simulink library "THBCreator"  (Simulink 8.2)
settings: Solver=ode45  StartTime=0.0  StopTime=10.0  RelTol=1e-3
settings Model: Creator=lena.frank  LastModifiedBy=drhf

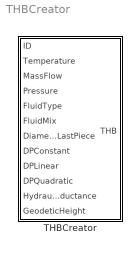
== system THBCreator ==
  THBCreator : Subsystem  InitFcn=load('THB.mat');  mask(THBCreator){Inport_ID=on, Inport_T=on, Inport_mdot=on, Inport_p=on, Inport_type=on, Inport_mix=on, Inport_d=on, Inport_c=on, Inport_l=on, Inport_q=on, Inport_LH=on, Inport_H=on, ID=20001, T=20, mdot=0, p=1e5, FluidType=1, FluidMix=0, d=0.01, c=0, l=0, q=0, LH=0, H=0, Annotation_ID=off, Annotation_T=off, Annotation_mdot=off, Annotation_p=off, Annotation_type=off, Annotation_mix=off, Annotation_d=off, Annotation_c=off, Annotation_l=off, Annotation_q=off, Annotation_LH=off, Annotation_H=off}
      mask prompts: Inport_ID "ID as inport"; Inport_T "temperature as inport"; Inport_mdot "mass flow rate as inport"; Inport_p "pressure as inport"; Inport_type "fluid type as inport"; Inport_mix "fluid mix as inport"; Inport_d "diameter last piece as inport"; Inport_c "constant pressure drop coefficient as inport"; Inport_l "linear pressure drop coefficient as inport"; Inport_q "quadratic pressure drop coefficient as inport"; Inport_LH "hydraulic inductance as inport"; Inport_H "geodetic height as inport"; ID "ID [1]"; T "temperature [°C]"; mdot "mass flow rate [kg/s]"; p "pressure [Pa]"; FluidType "fluid type [enum]"; FluidMix "fluid mix [1]"; d "diameter last piece [m]"; c "constant pressure drop coefficient [Pa]"; l "linear pressure drop coefficient [Pa/(kg/s)]"; q "quadratic pressure drop coefficient [Pa/(kg/s)²]"; LH "hydraulic inductance [1/m]"; H "geodetic height"; Annotation_ID "ID as annotation"; Annotation_T "temperature as annotation"; Annotation_mdot "mass flow rate as annotation"; Annotation_p "pressure as annotation"; Annotation_type "fluid type as annotation"; Annotation_mix "fluid mix as annotation"; Annotation_d "diameter last piece as annotation"; Annotation_c "constant pressure drop coefficient as annotation"; Annotation_l "linear pressure drop coefficient as annotation"; Annotation_q "quadratic pressure drop coefficient as annotation"; Annotation_LH "hydraulic inductance as annotation"; Annotation_H "geodetic height as annotation"
      mask help: This block creates a THB from input signals.
      mask init:
      | MaskValue = get_param(gcb,'MaskValues');
      |     
      | if strcmp(MaskValue{1},'on') %ID
      |     if ~strcmp(get_param([gcb,'/ID'],'BlockType'),'Inport')
      |         delete_line(gcb,'ID/1','BusCreator/1'); %delete connection
      |         delete_block([gcb,'/ID']); %delete block
      |         add_block('built-in/Inport',[gcb,'/ID']); %add new block
      |         set_param([gcb, '/ID'],'Position',[50   1*50+8   50+30   1*50+8+14]); %set new block's position
      |         add_line(gcb,'ID/1','BusCreator/1'); %add new connection
      |         handles=get_param([gcb, '/ID'],'LineHandles'); %get line handles
      |         set(handles.Outport(1),'Name','ID'); %set line name
      |     end
      | else
      |     if ~strcmp(get_param([gcb,'/ID'],'BlockType'),'Constant')
      |         delete_line(gcb,'ID/1','BusCreator/1'); %delete connection
      |         delete_block([gcb,'/ID']); %delete block
      |         add_block('built-in/Constant',[gcb,'/ID']); %add new block
      |         set_param([gcb, '/ID'],'Position',[50   1*50   50+30   1*50+30]); %set new block's position
      |         set_param([gcb, '/ID'],'Value','ID'); %set mask varible as value
      |         add_line(gcb,'ID/1','BusCreator/1'); %add new connection
      |         handles=get_param([gcb, '/ID'],'LineHandles'); %get line handles
      |         set(handles.Outport(1),'Name','ID'); %set line name
      |     end
      | end
      | 
      | if strcmp(MaskValue{2},'on') %T
      |     if ~strcmp(get_param([gcb,'/Temperature'],'BlockType'),'Inport')
      |         delete_line(gcb,'Temperature/1','BusCreator/2'); %delete connection
      |         delete_block([gcb,'/Temperature']); %delete block
      |         add_block('built-in/Inport',[gcb,'/Temperature']); %add new block
      |         set_param([gcb, '/Temperature'],'Position',[50   2*50+8   50+30   2*50+8+14]); %set new block's position
      |         add_line(gcb,'Temperature/1','BusCreator/2'); %add new connection
      |         handles=get_param([gcb, '/Temperature'],'LineHandles'); %get line handles
      |         set(handles.Outport(1),'Name','Temperature'); %set line name
      |     end
      | else
      |     if ~strcmp(get_param([gcb,'/Temperature'],'BlockType'),'Constant')
      |         delete_line(gcb,'Temperature/1','BusCreator/2'); %delete connection
      |         delete_block([gcb,'/Temperature']); %delete block
      |         add_block('built-in/Constant',[gcb,'/Temperature']); %add new block
      |         set_param([gcb, '/Temperature'],'Position',[50   2*50   50+30   2*50+30]); %set new block's position
      |         set_param([gcb, '/Temperature'],'Value','T'); %set mask varible as value
      |         add_line(gcb,'Temperature/1','BusCreator/2'); %add new connection
      |         handles=get_param([gcb, '/Temperature'],'LineHandles'); %get line handles
      |         set(handles.Outport(1),'Name','Temperature'); %set line name
      |     end
      | end
      | 
      | if strcmp(MaskValue{3},'on') %MassFlow
      |     if ~strcmp(get_param([gcb,'/MassFlow'],'BlockType'),'Inport')
      |         delete_line(gcb,'MassFlow/1','BusCreator/3'); %delete connection
      |         delete_block([gcb,'/MassFlow']); %delete block
      |         add_block('built-in/Inport',[gcb,'/MassFlow']); %add new block
      |         set_param([gcb, '/MassFlow'],'Position',[50   3*50+8   50+30   3*50+8+14]); %set new block's position
      |         add_line(gcb,'MassFlow/1','BusCreator/3'); %add new connection
      |         handles=get_param([gcb, '/MassFlow'],'LineHandles'); %get line handles
      |         set(handles.Outport(1),'Name','MassFlow'); %set line name
      |     end
      | else
      |     if ~strcmp(get_param([gcb,'/MassFlow'],'BlockType'),'Constant')
      |         delete_line(gcb,'MassFlow/1','BusCreator/3'); %delete connection
      |         delete_block([gcb,'/MassFlow']); %delete block
      |         add_block('built-in/Constant',[gcb,'/MassFlow']); %add new block
      |         set_param([gcb, '/MassFlow'],'Position',[50   3*50   50+30   3*50+30]); %set new block's position
      |         set_param([gcb, '/MassFlow'],'Value','mdot'); %set mask varible as value
      |         add_line(gcb,'MassFlow/1','BusCreator/3'); %add new connection
      |         handles=get_param([gcb, '/MassFlow'],'LineHandles'); %get line handles
      |         set(handles.Outport(1),'Name','MassFlow'); %set line name
      |     end
      | end
      | 
      | if strcmp(MaskValue{4},'on') %Pressure
      |     if ~strcmp(get_param([gcb,'/Pressure'],'BlockType'),'Inport')
      |         delete_line(gcb,'Pressure/1','BusCreator/4'); %delete connection
      |         delete_block([gcb,'/Pressure']); %delete block
      |         add_block('built-in/Inport',[gcb,'/Pressure']); %add new block
      |         set_param([gcb, '/Pressure'],'Position',[50   4*50+8   50+30   4*50+8+14]); %set new block's position
      |         add_line(gcb,'Pressure/1','BusCreator/4'); %add new connection
      |         handles=get_param([gcb, '/Pressure'],'LineHandles'); %get line handles
      |         set(handles.Outport(1),'Name','Pressure'); %set line name
      |     end
      | else
      |     if ~strcmp(get_param([gcb,'/Pressure'],'BlockType'),'Constant')
      |         delete_line(gcb,'Pressure/1','BusCreator/4'); %delete connection
      |         delete_block([gcb,'/Pressure']); %delete block
      |         add_block('built-in/Constant',[gcb,'/Pressure']); %add new block
      |         set_param([gcb, '/Pressure'],'Position',[50   4*50   50+30   4*50+30]); %set new block's position
      |         set_param([gcb, '/Pressure'],'Value','p'); %set mask varible as value
      |         add_line(gcb,'Pressure/1','BusCreator/4'); %add new connection
      |         handles=get_param([gcb, '/Pressure'],'LineHandles'); %get line handles
      |         set(handles.Outport(1),'Name','Pressure'); %set line name
      |     end
      | end
      | 
      | if strcmp(MaskValue{5},'on') %FluidType
      |     if ~strcmp(get_param([gcb,'/FluidType'],'BlockType'),'Inport')
      |         delete_line(gcb,'FluidType/1','BusCreator/5'); %delete connection
      |         delete_block([gcb,'/FluidType']); %delete block
      |         add_block('built-in/Inport',[gcb,'/FluidType']); %add new block
      |         set_param([gcb, '/FluidType'],'Position',[50   5*50+8   50+30   5*50+8+14]); %set new block's position
      |         add_line(gcb,'FluidType/1','BusCreator/5'); %add new connection
      |         handles=get_param([gcb, '/FluidType'],'LineHandles'); %get line handles
      |         set(handles.Outport(1),'Name','FluidType'); %set line name
      |     end
      | else
      |     if ~strcmp(get_param([gcb,'/FluidType'],'BlockType'),'Constant')
      |         delete_line(gcb,'FluidType/1','BusCreator/5'); %delete connection
      |         delete_block([gcb,'/FluidType']); %delete block
      |         add_block('built-in/Constant',[gcb,'/FluidType']); %add new block
      |         set_param([gcb, '/FluidType'],'Position',[50   5*50   50+30   5*50+30]); %set new block's position
      |         set_param([gcb, '/FluidType'],'Value','FluidType'); %set mask varible as value
      |         add_line(gcb,'FluidType/1','BusCreator/5'); %add new connection
      |         handles=get_param([gcb, '/FluidType'],'LineHandles'); %get line handles
      |         set(handles.Outport(1),'Name','FluidType'); %set line name
      |     end
      | end
      | 
      | if strcmp(MaskValue{6},'on') %FluidMix
      |     if ~strcmp(get_param([gcb,'/FluidMix'],'BlockType'),'Inport')
      |         delete_line(gcb,'FluidMix/1','BusCreator/6'); %delete connection
      |         delete_block([gcb,'/FluidMix']); %delete block
      |         add_block('built-in/Inport',[gcb,'/FluidMix']); %add new block
      |         set_param([gcb, '/FluidMix'],'Position',[50   6*50+8   50+30   6*50+8+14]); %set new block's position
      |         add_line(gcb,'FluidMix/1','BusCreator/6'); %add new connection
      |         handles=get_param([gcb, '/FluidMix'],'LineHandles'); %get line handles
      |         set(handles.Outport(1),'Name','FluidMix'); %set line name
      |     end
      | else
      |     if ~strcmp(get_param([gcb,'/FluidMix'],'BlockType'),'Constant')
      |         delete_line(gcb,'FluidMix/1','BusCreator/6'); %delete connection
      |         delete_block([gcb,'/FluidMix']); %delete block
      |         add_block('built-in/Constant',[gcb,'/FluidMix']); %add new block
      |         set_param([gcb, '/FluidMix'],'Position',[50   6*50   50+30   6*50+30]); %set new block's position
      |         set_param([gcb, '/FluidMix'],'Value','FluidMix'); %set mask varible as value
      |         add_line(gcb,'FluidMix/1','BusCreator/6'); %add new connection
      |         handles=get_param([gcb, '/FluidMix'],'LineHandles'); %get line handles
      |         set(handles.Outport(1),'Name','FluidMix'); %set line name
      |     end
      | end
      | 
      | if strcmp(MaskValue{7},'on') %DiameterLastPiece
      |     if ~strcmp(get_param([gcb,'/DiameterLastPiece'],'BlockType'),'Inport')
      |         delete_line(gcb,'DiameterLastPiece/1','BusCreator/7'); %delete connection
      |         delete_block([gcb,'/DiameterLastPiece']); %delete block
      |         add_block('built-in/Inport',[gcb,'/DiameterLastPiece']); %add new block
      |         set_param([gcb, '/DiameterLastPiece'],'Position',[50   7*50+8   50+30   7*50+8+14]); %set new block's position
      |         add_line(gcb,'DiameterLastPiece/1','BusCreator/7'); %add new connection
      |         handles=get_param([gcb, '/DiameterLastPiece'],'LineHandles'); %get line handles
      |         set(handles.Outport(1),'Name','DiameterLastPiece'); %set line name
      |     end
      | else
      |     if ~strcmp(get_param([gcb,'/DiameterLastPiece'],'BlockType'),'Constant')
      |         delete_line(gcb,'DiameterLastPiece/1','BusCreator/7'); %delete connection
      |         delete_block([gcb,'/DiameterLastPiece']); %delete block
      |         add_block('built-in/Constant',[gcb,'/DiameterLastPiece']); %add new block
      |         set_param([gcb, '/DiameterLastPiece'],'Position',[50   7*50   50+30   7*50+30]); %set new block's position
      |         set_param([gcb, '/DiameterLastPiece'],'Value','d'); %set mask varible as value
      |         add_line(gcb,'DiameterLastPiece/1','BusCreator/7'); %add new connection
      |         handles=get_param([gcb, '/DiameterLastPiece'],'LineHandles'); %get line handles
      |         set(handles.Outport(1),'Name','DiameterLastPiece'); %set line name
      |     end
      | end
      | 
      | if strcmp(MaskValue{8},'on') %DPConstant
      |     if ~strcmp(get_param([gcb,'/DPConstant'],'BlockType'),'Inport')
      |         delete_line(gcb,'DPConstant/1','BusCreator/8'); %delete connection
      |         delete_block([gcb,'/DPConstant']); %delete block
      |         add_block('built-in/Inport',[gcb,'/DPConstant']); %add new block
      |         set_param([gcb, '/DPConstant'],'Position',[50   8*50+8   50+30   8*50+8+14]); %set new block's position
      |         add_line(gcb,'DPConstant/1','BusCreator/8'); %add new connection
      |         handles=get_param([gcb, '/DPConstant'],'LineHandles'); %get line handles
      |         set(handles.Outport(1),'Name','DPConstant'); %set line name
      |     end
      | else
      |     if ~strcmp(get_param([gcb,'/DPConstant'],'BlockType'),'Constant')
      |         delete_line(gcb,'DPConstant/1','BusCreator/8'); %delete connection
      |         delete_block([gcb,'/DPConstant']); %delete block
      |         add_block('built-in/Constant',[gcb,'/DPConstant']); %add new block
      |         set_param([gcb, '/DPConstant'],'Position',[50   8*50   50+30   8*50+30]); %set new block's position
      |         set_param([gcb, '/DPConstant'],'Value','c'); %set mask varible as value
      |         add_line(gcb,'DPConstant/1','BusCreator/8'); %add new connection
      |         handles=get_param([gcb, '/DPConstant'],'LineHandles'); %get line handles
      |         set(handles.Outport(1),'Name','DPConstant'); %set line name
      |     end
      | end
      | 
      | if strcmp(MaskValue{9},'on') %DPLinear
      |     if ~strcmp(get_param([gcb,'/DPLinear'],'BlockType'),'Inport')
      |         delete_line(gcb,'DPLinear/1','BusCreator/9'); %delete connection
      |         delete_block([gcb,'/DPLinear']); %delete block
      |         add_block('built-in/Inport',[gcb,'/DPLinear']); %add new block
      |         set_param([gcb, '/DPLinear'],'Position',[50   9*50+8   50+30   9*50+8+14]); %set new block's position
      |         add_line(gcb,'DPLinear/1','BusCreator/9'); %add new connection
      |         handles=get_param([gcb, '/DPLinear'],'LineHandles'); %get line handles
      |         set(handles.Outport(1),'Name','DPLinear'); %set line name
      |     end
      | else
      |     if ~strcmp(get_param([gcb,'/DPLinear'],'BlockType'),'Constant')
      |         delete_line(gcb,'DPLinear/1','BusCreator/9'); %delete connection
      |         delete_block([gcb,'/DPLinear']); %delete block
      |         add_block('built-in/Constant',[gcb,'/DPLinear']); %add new block
      |         set_param([gcb, '/DPLinear'],'Position',[50   9*50   50+30   9*50+30]); %set new block's position
      |         set_param([gcb, '/DPLinear'],'Value','l'); %set mask varible as value
      |         add_line(gcb,'DPLinear/1','BusCreator/9'); %add new connection
      |         handles=get_param([gcb, '/DPLinear'],'LineHandles'); %get line handles
      |         set(handles.Outport(1),'Name','DPLinear'); %set line name
      |     end
      | end
      | 
      | if strcmp(MaskValue{10},'on') %DPQuadratic
      |     if ~strcmp(get_param([gcb,'/DPQuadratic'],'BlockType'),'Inport')
      |         delete_line(gcb,'DPQuadratic/1','BusCreator/10'); %delete connection
      |         delete_block([gcb,'/DPQuadratic']); %delete block
      |         add_block('built-in/Inport',[gcb,'/DPQuadratic']); %add new block
      |         set_param([gcb, '/DPQuadratic'],'Position',[50   10*50+8   50+30   10*50+8+14]); %set new block's position
      |         add_line(gcb,'DPQuadratic/1','BusCreator/10'); %add new connection
      |         handles=get_param([gcb, '/DPQuadratic'],'LineHandles'); %get line handles
      |         set(handles.Outport(1),'Name','DPQuadratic'); %set line name
      |     end
      | else
      |     if ~strcmp(get_param([gcb,'/DPQuadratic'],'BlockType'),'Constant')
      |         delete_line(gcb,'DPQuadratic/1','BusCreator/10'); %delete connection
      |         delete_block([gcb,'/DPQuadratic']); %delete block
      |         add_block('built-in/Constant',[gcb,'/DPQuadratic']); %add new block
      |         set_param([gcb, '/DPQuadratic'],'Position',[50   10*50   50+30   10*50+30]); %set new block's position
      |         set_param([gcb, '/DPQuadratic'],'Value','q'); %set mask varible as value
      |         add_line(gcb,'DPQuadratic/1','BusCreator/10'); %add new connection
      |         handles=get_param([gcb, '/DPQuadratic'],'LineHandles'); %get line handles
      |         set(handles.Outport(1),'Name','DPQuadratic'); %set line name
      |     end
      | end
      | 
      | if strcmp(MaskValue{11},'on') %HydraulicInductance
      |     if ~strcmp(get_param([gcb,'/HydraulicInductance'],'BlockType'),'Inport')
      |         delete_line(gcb,'HydraulicInductance/1','BusCreator/11'); %delete connection
      |         delete_block([gcb,'/HydraulicInductance']); %delete block
      |         add_block('built-in/Inport',[gcb,'/HydraulicInductance']); %add new block
      |         set_param([gcb, '/HydraulicInductance'],'Position',[50   11*50+8   50+30   11*50+8+14]); %set new block's position
      |         add_line(gcb,'HydraulicInductance/1','BusCreator/11'); %add new connection
      |         handles=get_param([gcb, '/HydraulicInductance'],'LineHandles'); %get line handles
      |         set(handles.Outport(1),'Name','HydraulicInductance'); %set line name
      |     end
      | else
      |     if ~strcmp(get_param([gcb,'/HydraulicInductance'],'BlockType'),'Constant')
      |         delete_line(gcb,'HydraulicInductance/1','BusCreator/11'); %delete connection
      |         delete_block([gcb,'/HydraulicInductance']); %delete block
      |         add_block('built-in/Constant',[gcb,'/HydraulicInductance']); %add new block
      |         set_param([gcb, '/HydraulicInductance'],'Position',[50   11*50   50+30   11*50+30]); %set new block's position
      |         set_param([gcb, '/HydraulicInductance'],'Value','LH'); %set mask varible as value
      |         add_line(gcb,'HydraulicInductance/1','BusCreator/11'); %add new connection
      |         handles=get_param([gcb, '/HydraulicInductance'],'LineHandles'); %get line handles
      |         set(handles.Outport(1),'Name','HydraulicInductance'); %set line name
      |     end
      | end
      | 
      | if strcmp(MaskValue{12},'on') %GeodeticHeight
      |     if ~strcmp(get_param([gcb,'/GeodeticHeight'],'BlockType'),'Inport')
      |         delete_line(gcb,'GeodeticHeight/1','BusCreator/12'); %delete connection
      |         delete_block([gcb,'/GeodeticHeight']); %delete block
      |         add_block('built-in/Inport',[gcb,'/GeodeticHeight']); %add new block
      |         set_param([gcb, '/GeodeticHeight'],'Position',[50   12*50+8   50+30   12*50+8+14]); %set new block's position
      |         add_line(gcb,'GeodeticHeight/1','BusCreator/12'); %add new connection
      |         handles=get_param([gcb, '/GeodeticHeight'],'LineHandles'); %get line handles
      |         set(handles.Outport(1),'Name','GeodeticHeight'); %set line name
      |     end
      | else
      |     if ~strcmp(get_param([gcb,'/GeodeticHeight'],'BlockType'),'Constant')
      |         delete_line(gcb,'GeodeticHeight/1','BusCreator/12'); %delete connection
      |         delete_block([gcb,'/GeodeticHeight']); %delete block
      |         add_block('built-in/Constant',[gcb,'/GeodeticHeight']); %add new block
      |         set_param([gcb, '/GeodeticHeight'],'Position',[50   12*50   50+30   12*50+30]); %set new block's position
      |         set_param([gcb, '/GeodeticHeight'],'Value','H'); %set mask varible as value
      |         add_line(gcb,'GeodeticHeight/1','BusCreator/12'); %add new connection
      |         handles=get_param([gcb, '/GeodeticHeight'],'LineHandles'); %get line handles
      |         set(handles.Outport(1),'Name','GeodeticHeight'); %set line name
      |     end
      | end
      mask Help:
      | web('THBCreator.html','-helpbrowser'
      | web(fullfile(path_carnot('help'),'THBCreator.html'),'-helpbrowser')
      mask Callback Inport_ID: THBCreator_ParamCallback;
      mask Callback Inport_T: THBCreator_ParamCallback;
      mask Callback Inport_mdot: THBCreator_ParamCallback;
      mask Callback Inport_p: THBCreator_ParamCallback;
      mask Callback Inport_type: THBCreator_ParamCallback;
      mask Callback Inport_mix: THBCreator_ParamCallback;
      mask Callback Inport_d: THBCreator_ParamCallback;
      mask Callback Inport_c: THBCreator_ParamCallback;
      mask Callback Inport_l: THBCreator_ParamCallback;
      mask Callback Inport_q: THBCreator_ParamCallback;
      mask Callback Inport_LH: THBCreator_ParamCallback;
      mask Callback Inport_H: THBCreator_ParamCallback;
      mask Callback Annotation_ID: THBCreator_ParamCallback;
      mask Callback Annotation_T: THBCreator_ParamCallback;
      mask Callback Annotation_mdot: THBCreator_ParamCallback;
      mask Callback Annotation_p: THBCreator_ParamCallback;
      mask Callback Annotation_type: THBCreator_ParamCallback;
      mask Callback Annotation_mix: THBCreator_ParamCallback;
      mask Callback Annotation_d: THBCreator_ParamCallback;
      mask Callback Annotation_c: THBCreator_ParamCallback;
      mask Callback Annotation_l: THBCreator_ParamCallback;
      mask Callback Annotation_q: THBCreator_ParamCallback;
      mask Callback Annotation_LH: THBCreator_ParamCallback;
      mask Callback Annotation_H: THBCreator_ParamCallback;

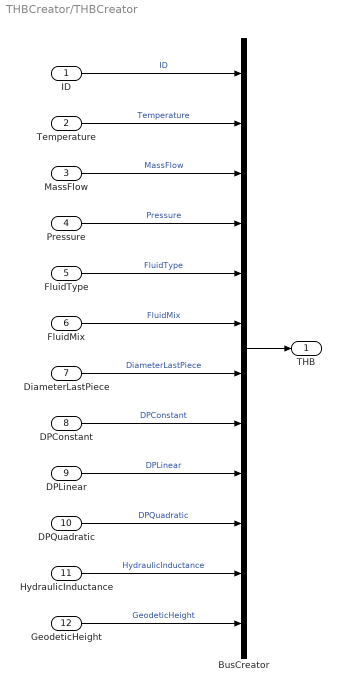
== system THBCreator/THBCreator ==
  ID : Inport
  Temperature : Inport  Port=2
  MassFlow : Inport  Port=3
  Pressure : Inport  Port=4
  FluidType : Inport  Port=5
  FluidMix : Inport  Port=6
  DiameterLastPiece : Inport  Port=7
  DPConstant : Inport  Port=8
  DPLinear : Inport  Port=9
  DPQuadratic : Inport  Port=10
  HydraulicInductance : Inport  Port=11
  GeodeticHeight : Inport  Port=12
  BusCreator : BusCreator  Inputs=12  OutDataTypeStr=Bus: THB
  THB : Outport
  wires:
  GeodeticHeight/1 -> BusCreator/12  "GeodeticHeight"
  HydraulicInductance/1 -> BusCreator/11  "HydraulicInductance"
  DPQuadratic/1 -> BusCreator/10  "DPQuadratic"
  DPLinear/1 -> BusCreator/9  "DPLinear"
  DPConstant/1 -> BusCreator/8  "DPConstant"
  DiameterLastPiece/1 -> BusCreator/7  "DiameterLastPiece"
  FluidMix/1 -> BusCreator/6  "FluidMix"
  FluidType/1 -> BusCreator/5  "FluidType"
  Pressure/1 -> BusCreator/4  "Pressure"
  MassFlow/1 -> BusCreator/3  "MassFlow"
  Temperature/1 -> BusCreator/2  "Temperature"
  ID/1 -> BusCreator/1  "ID"
  BusCreator/1 -> THB/1
